simulink model "clutch_model"  (R2021a)
settings: Solver=VariableStepAuto  StartTime=0.0  StopTime=1  RelTol=1e-3
settings Model: Creator=Cal  LastModifiedBy=Cal

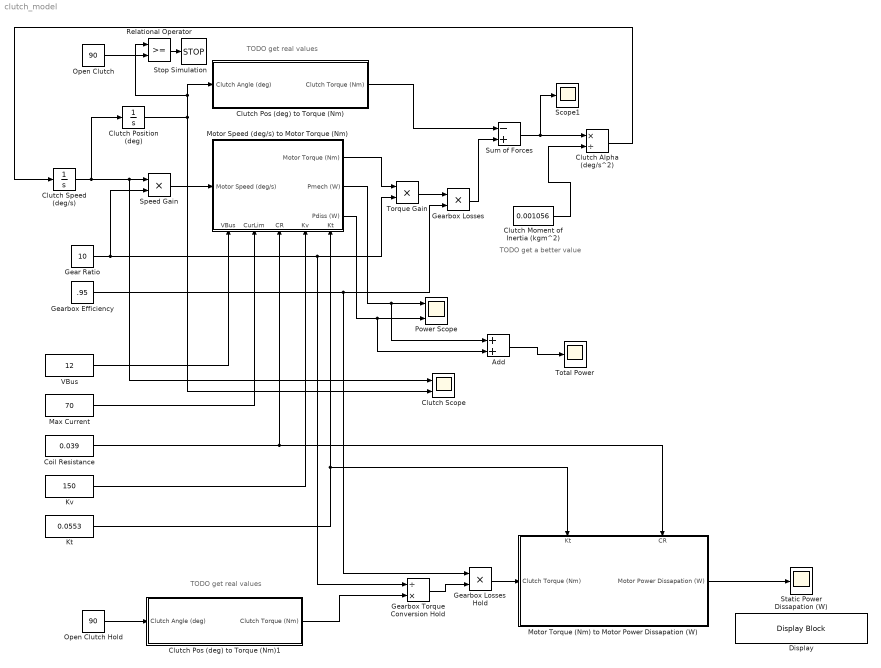
== system clutch_model ==
  note: TODO get real values
  note: TODO get a better value
  note: TODO get real values
  Add : Sum
  Clutch Alpha (deg/s^2) : Product  Inputs=*/
  Clutch Moment of Inertia (kgm^2) : Constant  Value=0.001056
  Clutch Pos (deg) to Torque (Nm) : Subsystem
  Clutch Pos (deg) to Torque (Nm)1 : Subsystem
  Clutch Position (deg) : Integrator
  Clutch Scope : Scope  NumInputPorts=2
  Clutch Speed (deg/s) : Integrator
  Coil Resistance : Constant  Value=0.039
  Display : DisplayBlock  LabelPosition=Hide  Format=short  Transparency=1
  Gear Ratio : Constant  Value=10
  Gearbox Efficiency : Constant  Value=.95
  Gearbox Losses : Product
  Gearbox Losses Hold : Product
  Gearbox Torque Conversion Hold : Product  Inputs=/*
  Kt : Constant  Value=0.0553
  Kv : Constant  Value=150
  Max Current : Constant  Value=70
  Motor Speed (deg/s) to Motor Torque (Nm) : Subsystem
      settings: PortSchema="{\"entries\":[{\"content\":{\"sides\":[{\"content\":{\"connectorIds\":[\"In1\"]},\"type\":\"ConnectorPlacement.EquallySpacedRectSide\",\"uuid\":\"7e3d6259-f020-48d4-ab2f-cc02f3e205f3\"},{\"content\":{\"connectorIds\":[\"Out1\",\"Out2\",\"Out3\"],\"side\":\"RIGHT\"},\"type\":\"ConnectorPlacement.EquallySpacedRectSide\",\"uuid\":\"df711253-8a83-44a2-b4f6-36021a4fbdad\"},{\"content\":{\"connectorIds\":[],\"side\":\"TOP\"},\"type\":\"ConnectorPlacement.EquallySpacedRectSide\",\"uuid\":\"808ed9f2-c99b-45a4-8d17-90091b6202b6\"},{\"content\":{\"connectorIds\":[\"In2\",\"In3\",\"In4\",\"In5\",\"In6\"],\"side\":\"BOTTOM\"},\"type\":\"ConnectorPlacement.EquallySpacedRectSide\",\"uuid\":\"e83684b7-d3eb-4f08-87c8-e935429af94a\"}]},\"type\":\"ConnectorPlacement.EquallySpacedConnector\",\"uuid\":\"e9285cd7-c097-4ff9-90f5-d18f52844aac\"}],\"packageUris\":[\"http://schema.mathworks.com/mf0/Connector/R2020b\"],\"version\":\"1.0\"}"
  Motor Torque (Nm) to Motor Power Dissapation (W) : Subsystem
      settings: PortSchema="{\"entries\":[{\"content\":{\"sides\":[{\"content\":{\"connectorIds\":[\"In1\"]},\"type\":\"ConnectorPlacement.EquallySpacedRectSide\",\"uuid\":\"3ec64108-34b1-4214-af14-de7d9a6b89d7\"},{\"content\":{\"connectorIds\":[\"Out1\"],\"side\":\"RIGHT\"},\"type\":\"ConnectorPlacement.EquallySpacedRectSide\",\"uuid\":\"a66a176f-0d37-451a-b520-e1afd774ae54\"},{\"content\":{\"connectorIds\":[\"In2\",\"In3\"],\"side\":\"TOP\"},\"type\":\"ConnectorPlacement.EquallySpacedRectSide\",\"uuid\":\"ac2b7dd3-1c21-45f4-ac26-7b034153dae5\"}]},\"type\":\"ConnectorPlacement.EquallySpacedConnector\",\"uuid\":\"9fe287c7-b94b-4824-b10a-73f55dfd2ff0\"}],\"packageUris\":[\"http://schema.mathworks.com/mf0/Connector/R2020b\"],\"version\":\"1.0\"}"
  Open Clutch : Constant  Value=90
  Open Clutch Hold : Constant  Value=90
  Power Scope : Scope  NumInputPorts=2
  Relational Operator : RelationalOperator  OutDataTypeStr=boolean  RndMeth=Simplest
  Scope1 : Scope
  Speed Gain : Product
  Static Power Dissapation (W) : Scope
  Stop Simulation : Stop
  Sum of Forces : Sum  Inputs=-+
  Torque Gain : Product
  Total Power : Scope
  VBus : Constant  Value=12
  wires:
  Clutch Speed (deg/s)/1 -> Clutch Scope/1, Speed Gain/1, Clutch Position (deg)/1
  Clutch Position (deg)/1 -> Clutch Scope/2, Relational Operator/1, Clutch Pos (deg) to Torque (Nm)/1(Clutch Angle (deg))
  Speed Gain/1 -> Motor Speed (deg/s) to Motor Torque (Nm)/1(Motor Speed (deg/s))
  Clutch Pos (deg) to Torque (Nm)/1(Clutch Torque (Nm)) -> Sum of Forces/1
  Motor Speed (deg/s) to Motor Torque (Nm)/1(Motor Torque (Nm)) -> Torque Gain/1
  Torque Gain/1 -> Gearbox Losses/1
  Gearbox Losses/1 -> Sum of Forces/2
  Sum of Forces/1 -> Scope1/1, Clutch Alpha (deg/s^2)/1
  Clutch Moment of Inertia (kgm^2)/1 -> Clutch Alpha (deg/s^2)/2
  Clutch Alpha (deg/s^2)/1 -> Clutch Speed (deg/s)/1
  Gear Ratio/1 -> Speed Gain/2, Gearbox Torque Conversion Hold/1, Torque Gain/2
  VBus/1 -> Motor Speed (deg/s) to Motor Torque (Nm)/2(VBus)
  Coil Resistance/1 -> Motor Torque (Nm) to Motor Power Dissapation (W)/3(CR), Motor Speed (deg/s) to Motor Torque (Nm)/4(CR)
  Kv/1 -> Motor Speed (deg/s) to Motor Torque (Nm)/5(Kv)
  Kt/1 -> Motor Torque (Nm) to Motor Power Dissapation (W)/2(Kt), Motor Speed (deg/s) to Motor Torque (Nm)/6(Kt)
  Gearbox Efficiency/1 -> Gearbox Losses Hold/1, Gearbox Losses/2
  Open Clutch/1 -> Relational Operator/2
  Relational Operator/1 -> Stop Simulation/1
  Motor Speed (deg/s) to Motor Torque (Nm)/3(Pdiss (W)) -> Add/2, Power Scope/2
  Max Current/1 -> Motor Speed (deg/s) to Motor Torque (Nm)/3(CurLim)
  Motor Speed (deg/s) to Motor Torque (Nm)/2(Pmech (W)) -> Add/1, Power Scope/1
  Add/1 -> Total Power/1
  Open Clutch Hold/1 -> Clutch Pos (deg) to Torque (Nm)1/1(Clutch Angle (deg))
  Clutch Pos (deg) to Torque (Nm)1/1(Clutch Torque (Nm)) -> Gearbox Torque Conversion Hold/2
  Gearbox Torque Conversion Hold/1 -> Gearbox Losses Hold/2
  Gearbox Losses Hold/1 -> Motor Torque (Nm) to Motor Power Dissapation (W)/1(Clutch Torque (Nm))
  Motor Torque (Nm) to Motor Power Dissapation (W)/1(Motor Power Dissapation (W)) -> Static Power Dissapation (W)/1

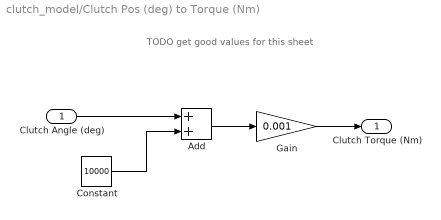
== system clutch_model/Clutch Pos (deg) to Torque (Nm) ==
  note: TODO get good values for this sheet
  Clutch Angle (deg) : Inport
  Add : Sum
  Constant : Constant  Value=10000
  Gain : Gain  Gain=0.001
  Clutch Torque (Nm) : Outport
  wires:
  Clutch Angle (deg)/1 -> Add/1
  Add/1 -> Gain/1
  Gain/1 -> Clutch Torque (Nm)/1
  Constant/1 -> Add/2

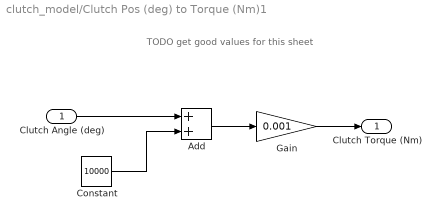
== system clutch_model/Clutch Pos (deg) to Torque (Nm)1 ==
  note: TODO get good values for this sheet
  Clutch Angle (deg) : Inport
  Add : Sum
  Constant : Constant  Value=10000
  Gain : Gain  Gain=0.001
  Clutch Torque (Nm) : Outport
  wires:
  Clutch Angle (deg)/1 -> Add/1
  Add/1 -> Gain/1
  Gain/1 -> Clutch Torque (Nm)/1
  Constant/1 -> Add/2

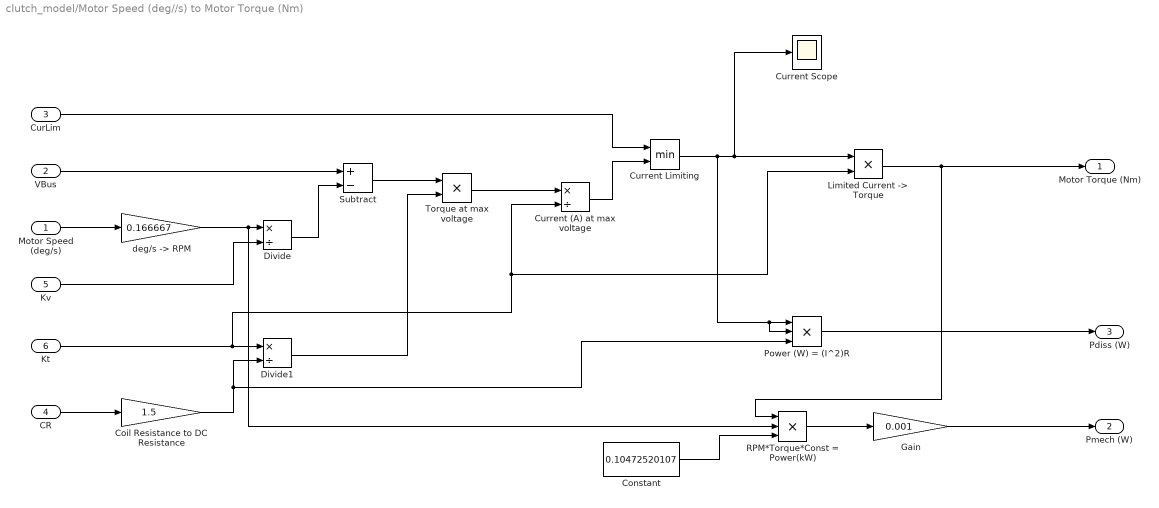
== system clutch_model/Motor Speed (deg//s) to Motor Torque (Nm) ==
  Motor Speed (deg/s) : Inport
  VBus : Inport  Port=2
  CurLim : Inport  Port=3
  CR : Inport  Port=4
  Kv : Inport  Port=5
  Kt : Inport  Port=6
  Coil Resistance to DC Resistance : Gain  Gain=1.5
  Constant : Constant  Value=0.10472520107
  Current (A) at max voltage : Product  Inputs=*/
  Current Limiting : MinMax  Inputs=2
  Current Scope : Scope
  Divide : Product  Inputs=*/
  Divide1 : Product  Inputs=*/
  Gain : Gain  Gain=0.001
  "Limited Current -> Torque" : Product
  Power (W) = (I^2)R : Product  Inputs=3
  RPM*Torque*Const = Power(kW) : Product  Inputs=3
  Subtract : Sum  Inputs=+-
  Torque at max voltage : Product
  "deg/s -> RPM" : Gain  Gain=0.166667
  Motor Torque (Nm) : Outport
  Pmech (W) : Outport  Port=2
  Pdiss (W) : Outport  Port=3
  wires:
  Motor Speed (deg/s)/1 -> "deg/s -> RPM"/1
  CR/1 -> Coil Resistance to DC Resistance/1
  "deg/s -> RPM"/1 -> RPM*Torque*Const = Power(kW)/2, Divide/1
  Kv/1 -> Divide/2
  VBus/1 -> Subtract/1
  Divide/1 -> Subtract/2
  Kt/1 -> "Limited Current -> Torque"/2, Current (A) at max voltage/2, Divide1/1
  Coil Resistance to DC Resistance/1 -> Power (W) = (I^2)R/3, Divide1/2
  Divide1/1 -> Torque at max voltage/2
  Subtract/1 -> Torque at max voltage/1
  Torque at max voltage/1 -> Current (A) at max voltage/1
  Constant/1 -> RPM*Torque*Const = Power(kW)/3
  RPM*Torque*Const = Power(kW)/1 -> Gain/1
  Gain/1 -> Pmech (W)/1
  Current Limiting/1 -> Power (W) = (I^2)R/2, Power (W) = (I^2)R/1, Current Scope/1, "Limited Current -> Torque"/1
  Power (W) = (I^2)R/1 -> Pdiss (W)/1
  CurLim/1 -> Current Limiting/1
  Current (A) at max voltage/1 -> Current Limiting/2
  "Limited Current -> Torque"/1 -> RPM*Torque*Const = Power(kW)/1, Motor Torque (Nm)/1

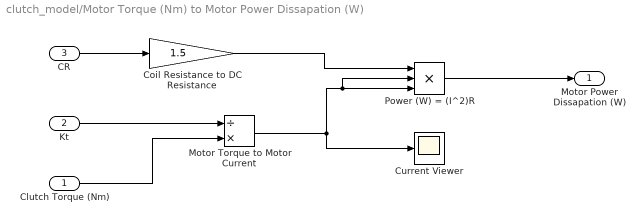
== system clutch_model/Motor Torque (Nm) to Motor Power Dissapation (W) ==
  Clutch Torque (Nm) : Inport
  Kt : Inport  Port=2
  CR : Inport  Port=3
  Coil Resistance to DC Resistance : Gain  Gain=1.5
  Current Viewer : Scope
  Motor Torque to Motor Current : Product  Inputs=/*
  Power (W) = (I^2)R : Product  Inputs=3
  Motor Power Dissapation (W) : Outport
  wires:
  CR/1 -> Coil Resistance to DC Resistance/1
  Kt/1 -> Motor Torque to Motor Current/1
  Clutch Torque (Nm)/1 -> Motor Torque to Motor Current/2
  Motor Torque to Motor Current/1 -> Current Viewer/1, Power (W) = (I^2)R/2, Power (W) = (I^2)R/3
  Coil Resistance to DC Resistance/1 -> Power (W) = (I^2)R/1
  Power (W) = (I^2)R/1 -> Motor Power Dissapation (W)/1
